simulink model "DCCONTROL_INDOMAIN"  (R2026a)
settings: Solver=VariableStepAuto
model workspace (MAT data in the model file):
  Kb = 0.01
  Kt = 0.01
values from neighbouring files (symbols this model uses):
  B = input('Input the Rotor rotational friction constant: ')    [scriptforDCCONTROL_INDOMAIN.m]
  Kd = 0    [scriptforDCCONTROL_INDOMAIN.m]
  Ki = 2 * (tau_m_baseline / tau_m)    [scriptforDCCONTROL_INDOMAIN.m]
  Kp = 3 * (tau_m_baseline / tau_m)    [scriptforDCCONTROL_INDOMAIN.m]
  omega_ref = input('Input the reference speed (rad/s) at which the motor should steady at: ')    [scriptforDCCONTROL_INDOMAIN.m]
  Ra = input('Input the Armature resistance: ')    [scriptforDCCONTROL_INDOMAIN.m]
  V_supply = input('Input the Voltage Supply: ')    [scriptforDCCONTROL_INDOMAIN.m]
libraries: fl_lib x10, nesl_utility x8, ee_lib x2
settings Model: Creator=Kratos  LastModifiedBy=Kratos

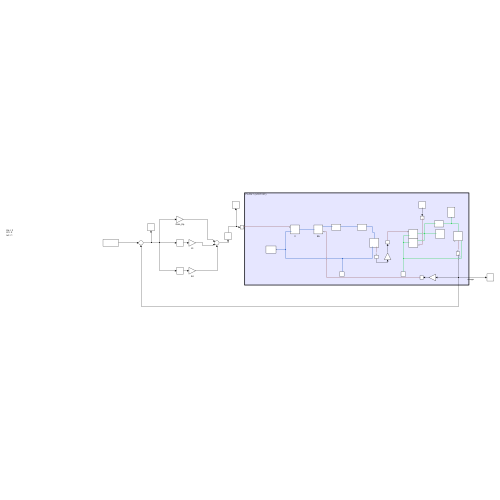
[thumbnail: Simulink's stored preview of the top-level diagram]
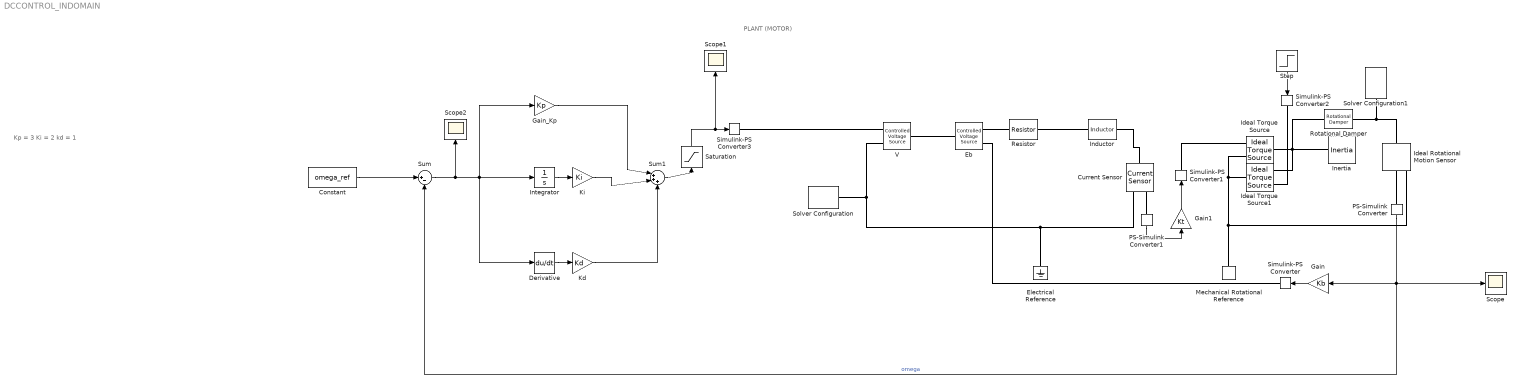
== system DCCONTROL_INDOMAIN ==
  note: Kp = 3
      | Ki = 2
      | kd = 1
  note: PLANT (MOTOR)
  Constant : Constant  Value=omega_ref
  Current Sensor : fl_lib/Electrical/Electrical Sensors/Current Sensor
  Derivative : Derivative
  Eb : fl_lib/Electrical/Electrical Sources/Controlled Voltage Source
  Electrical Reference : fl_lib/Electrical/Electrical Elements/Electrical Reference
  Gain : Gain  Gain=Kb
  Gain1 : Gain  Gain=Kt
  Gain_Kp : Gain  Gain=Kp
  Ideal Rotational Motion Sensor : fl_lib/Mechanical/Mechanical Sensors/Ideal Rotational Motion Sensor  reference=foundation.enum.MeasurementReference.difference  acceleration_port=false  velocity_port=true  position_port=true  wrap_angle=false  offset=0 rad
  Ideal Torque Source : fl_lib/Mechanical/Mechanical Sources/Ideal Torque Source
  Ideal Torque Source1 : fl_lib/Mechanical/Mechanical Sources/Ideal Torque Source
  Inductor : ee_lib/Passive/Inductor  l=La H  enable_L_tol=ee.enum.toleranceApplication.none  L_tol=20  tol_distribution=ee.enum.toleranceDistribution.uniform  nSigma=4  r=0 Ohm  g=1e-9 1/Ohm  enable_operating_limits=ee.enum.enable.no  operating_limit_action=ee.enum.passive.reportOpLim.warn  max_working_current=1 A  power_rating=1 W  i_L_specify=off  i_L_priority=High  i_L=0 A  i_L_nominal_specify=off  i_L_nominal_value=1  i_L_nominal_unit=A
  Inertia : fl_lib/Mechanical/Rotational Elements/Inertia  inertia=J kg*m^2  num_ports=foundation.enum.numPorts2.one  w_specify=off  w_priority=High  w=0 rad/s  w_nominal_specify=off  w_nominal_value=1  w_nominal_unit=rad/s  t_specify=off  t_priority=None  t=0 N*m  t_nominal_specify=off  t_nominal_value=1  t_nominal_unit=N*m
  Integrator : Integrator
  Kd : Gain  Gain=Kd
  Ki : Gain  Gain=Ki
  Mechanical Rotational Reference : fl_lib/Mechanical/Rotational Elements/Mechanical Rotational Reference
  PS-Simulink Converter : nesl_utility/PS-Simulink Converter  PhysicalDomain=network_engine_domain  SubClassName=ps_output  LeftPortType=input  RightPortType=output  PseudoPeriodic=off  Frequencies=[]  VectorFormat=inherit  Unit=inherit  AffineConversion=off
  PS-Simulink Converter1 : nesl_utility/PS-Simulink Converter  PhysicalDomain=network_engine_domain  SubClassName=ps_output  LeftPortType=input  RightPortType=output  PseudoPeriodic=off  Frequencies=[]  VectorFormat=inherit  Unit=inherit  AffineConversion=off
  Resistor : ee_lib/Passive/Resistor  R=Ra Ohm  enable_R_tol=ee.enum.toleranceApplication.none  R_tol=5  tol_distribution=ee.enum.toleranceDistribution.uniform  nSigma=4  enable_operating_limits=ee.enum.enable.no  operating_limit_action=ee.enum.passive.reportOpLim.warn  power_rating=1 W  max_working_voltage=100 V  noise_mode=ee.enum.sources.noise.Disabled  Tdevice=25 degC  sample_time=1e-3 s  repeatability=ee.enum.ic.repeatability.notRepeatable  user_seed=0  auto_seed=3499211588  power_derating_T1=70 degC  power_derating_T2=155 degC  operating_temperature_range_vec=[-50, 150] degC  alpha=3.93e-3 1/K  Tmeas=25 degC  thermal_mass=100 J/K  temperature_specify=off  temperature_priority=High  temperature=298.15 K  temperature_nominal_specify=off  temperature_nominal_value=1  temperature_nominal_unit=K
  Rotational Damper : fl_lib/Mechanical/Rotational Elements/Rotational Damper  D=B N*m*s/rad  w_specify=off  w_priority=None  w=0 rad/s  w_nominal_specify=off  w_nominal_value=1  w_nominal_unit=rad/s  t_specify=off  t_priority=None  t=0 N*m  t_nominal_specify=off  t_nominal_value=1  t_nominal_unit=N*m
  Saturation : Saturate  UpperLimit=V_supply  LowerLimit=0
  Scope : Scope
      settings: ActiveDisplayYMinimum=-2.0507072921680938  ActiveDisplayYMaximum=2.3567012339433933
  Scope1 : Scope
      settings: ActiveDisplayYMinimum=-0.51839532171290958  ActiveDisplayYMaximum=17.47792539567039
  Scope2 : Scope
      settings: ActiveDisplayYMinimum=-3.4827838106559259  ActiveDisplayYMaximum=15.413352942596536  DataLoggingVariableName=ScopeData2
  Simulink-PS Converter{,1..3} (4 alike) : nesl_utility/Simulink-PS Converter  PhysicalDomain=network_engine_domain  SubClassName=ps_input  LeftPortType=input  RightPortType=output  PseudoPeriodic=off  Frequencies=[]  NoiseDistribution=none  NoiseParameters=[]  Unit=1  AffineConversion=off  FilteringAndDerivatives=provide  SimscapeFilterOrder=1  InputFilterTimeConstant=0.001  UdotUserProvided=0
  Solver Configuration : nesl_utility/Solver Configuration  PhysicalDomain=network_engine_domain  SubClassName=solver  LeftPortType=input  RightPortType=generic  Tones=[]  Harmonics=[]  SimulateNoise=off  Profile=off  UseLocalSampling=off  EnableSwitchedLinearOptims=on  FrequencyDomain=off  UseCCode=off  RelTol=0.001  AbsTol=0.001  MinStep=1e-09  ToWorkspace=off  RevertToSquareIcSolve=off  NumHomotopyIterations=100  PhasorMode=off  PhasorModeNumHarmonics=1  ConsistencySolver=NEWTON_XTOL_AFTER_FTOL  CanonicalOrdering=CANONICAL  OptimizeIntermediates=OPTIMIZED  IndexReductionMethod=DerivativeReplacement  DoDC=off  ResidualTolerance=1e-09  ConsistencyTolSource=GLOBAL  ConsistencyAbsTol=0.001  ConsistencyRelTol=0.001  ConsistencyTolFactor=0.001  UseLocalSolver=off  LocalSolverChoice=NE_BACKWARD_EULER_ADVANCER  ResolveIndetEquations=on  FunctionEvalNumThread=1  LocalSolverSampleTime=0.001  DoFixedCost=off  MaxNonlinIter=3  MaxModeIter=2  ComputeImpulses=off  ImpulseIterations=2  LinearAlgebra=auto  LinearAlgebraNumThread=0  EquationFormulation=NE_TIME_EF  DelaysMemoryBudget=1024  AutomaticFiltering=on  FilteringTimeConstant=0.001  PartitionStorageMethod=AS_NEEDED  PartitionMemoryBudget=1024  PartitionMethod=ROBUST  MultibodyUseLocalSolver=off  MultibodyLocalSolverChoice=ODE1  MultibodyLocalSolverSampleTime=0.001
  Solver Configuration1 : nesl_utility/Solver Configuration  PhysicalDomain=network_engine_domain  SubClassName=solver  LeftPortType=input  RightPortType=generic  Tones=[]  Harmonics=[]  SimulateNoise=off  Profile=off  UseLocalSampling=off  EnableSwitchedLinearOptims=on  FrequencyDomain=off  UseCCode=off  RelTol=0.001  AbsTol=0.001  MinStep=1e-09  ToWorkspace=off  RevertToSquareIcSolve=off  NumHomotopyIterations=100  PhasorMode=off  PhasorModeNumHarmonics=1  ConsistencySolver=NEWTON_XTOL_AFTER_FTOL  CanonicalOrdering=CANONICAL  OptimizeIntermediates=OPTIMIZED  IndexReductionMethod=DerivativeReplacement  DoDC=off  ResidualTolerance=1e-09  ConsistencyTolSource=GLOBAL  ConsistencyAbsTol=0.001  ConsistencyRelTol=0.001  ConsistencyTolFactor=0.001  UseLocalSolver=off  LocalSolverChoice=NE_BACKWARD_EULER_ADVANCER  ResolveIndetEquations=on  FunctionEvalNumThread=1  LocalSolverSampleTime=0.001  DoFixedCost=off  MaxNonlinIter=3  MaxModeIter=2  ComputeImpulses=off  ImpulseIterations=2  LinearAlgebra=auto  LinearAlgebraNumThread=0  EquationFormulation=NE_TIME_EF  DelaysMemoryBudget=1024  AutomaticFiltering=on  FilteringTimeConstant=0.001  PartitionStorageMethod=AS_NEEDED  PartitionMemoryBudget=1024  PartitionMethod=ROBUST  MultibodyUseLocalSolver=off  MultibodyLocalSolverChoice=ODE1  MultibodyLocalSolverSampleTime=0.001
  Step : Step  Time=2  FinalValue=0.125  SampleTime=0
  Sum : Sum  Inputs=|+-
  Sum1 : Sum  Inputs=|+++
  V : fl_lib/Electrical/Electrical Sources/Controlled Voltage Source
  wires:
  PS-Simulink Converter/1 -> Scope/1, Sum/2, Gain/1  "omega"
  Gain/1 -> Simulink-PS Converter/1
  PS-Simulink Converter1/1 -> Gain1/1
  Gain1/1 -> Simulink-PS Converter1/1
  Step/1 -> Simulink-PS Converter2/1
  Constant/1 -> Sum/1
  Sum/1 -> Derivative/1, Gain_Kp/1, Integrator/1, Scope2/1
  Integrator/1 -> Ki/1
  Derivative/1 -> Kd/1
  Gain_Kp/1 -> Sum1/1
  Ki/1 -> Sum1/2
  Kd/1 -> Sum1/3
  Sum1/1 -> Saturation/1
  Saturation/1 -> Scope1/1, Simulink-PS Converter3/1
  connections:
  Inductor/LConn1 -- Resistor/RConn1
  V/LConn1 -- Eb/LConn1
  Eb/RConn2 -- Resistor/LConn1
  Current Sensor/RConn2 -- Electrical Reference/LConn1 -- V/RConn2 -- Solver Configuration/RConn1
  Inductor/RConn1 -- Current Sensor/LConn1
  Ideal Torque Source/LConn1 -- Inertia/LConn1 -- Ideal Torque Source1/RConn2 -- Rotational Damper/LConn1
  Rotational Damper/RConn1 -- Solver Configuration1/RConn1 -- Ideal Rotational Motion Sensor/LConn1
  Ideal Torque Source/RConn2 -- Ideal Torque Source1/LConn1 -- Ideal Rotational Motion Sensor/RConn1 -- Mechanical Rotational Reference/LConn1
  PS-Simulink Converter/LConn1 -- Ideal Rotational Motion Sensor/RConn2
  Simulink-PS Converter/RConn1 -- Eb/RConn1
  PS-Simulink Converter1/LConn1 -- Current Sensor/RConn1
  Simulink-PS Converter1/RConn1 -- Ideal Torque Source/RConn1
  Simulink-PS Converter2/RConn1 -- Ideal Torque Source1/RConn1
  Simulink-PS Converter3/RConn1 -- V/RConn1
